simulink model "Test_Memory_Block_Word_VRAM_Get_Pixel"  (Simulink 8.7)
settings: Solver=ode45  StartTime=0.0  StopTime=len  RelTol=1e-3
libraries: Miscellaneous x2, Memory_Blocks_Lib x1
settings Model: Creator=N  LastModifiedBy=Jozko Mrkvicka
settings DataIOCC: LimitDataPoints=off
settings DebuggingCC: UnderspecifiedInitializationDetection=Simplified  MergeDetectMultiDrivingBlocksExec=error
settings HardwareCC: ProdBitPerPointer=64  ProdLargestAtomicFloat=Float  ProdIntDivRoundTo=Zero  ProdEndianess=LittleEndian  ProdHWDeviceType=Intel->x86-64 (Windows64)
settings ModelReferenceCC: PropagateSignalLabelsOutOfModel=on

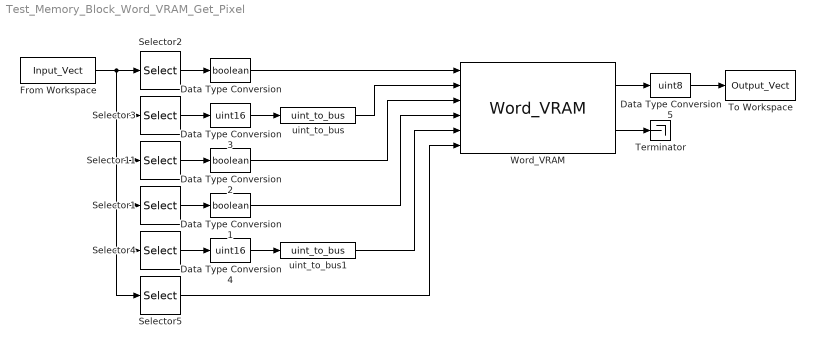
== system Test_Memory_Block_Word_VRAM_Get_Pixel ==
  Data Type Conversion : DataTypeConversion  OutDataTypeStr=boolean
  Data Type Conversion1 : DataTypeConversion  OutDataTypeStr=boolean
  Data Type Conversion2 : DataTypeConversion  OutDataTypeStr=boolean
  Data Type Conversion3 : DataTypeConversion  OutDataTypeStr=uint16
  Data Type Conversion4 : DataTypeConversion  OutDataTypeStr=uint16
  Data Type Conversion5 : DataTypeConversion  OutDataTypeStr=uint8
  From Workspace : FromWorkspace  VariableName=Input_Vect  SampleTime=1  Interpolate=off  OutputAfterFinalValue=Holding final value
  Selector1 : Selector  IndexMode=Zero-based  InputPortWidth=6  IndexOptions=Index vector (dialog)  Indices=3  OutputSizes=1
  Selector11 : Selector  IndexMode=Zero-based  InputPortWidth=6  IndexOptions=Index vector (dialog)  Indices=2  OutputSizes=1
  Selector2 : Selector  IndexMode=Zero-based  InputPortWidth=6  IndexOptions=Index vector (dialog)  Indices=0  OutputSizes=1
  Selector3 : Selector  IndexMode=Zero-based  InputPortWidth=6  IndexOptions=Index vector (dialog)  Indices=1  OutputSizes=1
  Selector4 : Selector  IndexMode=Zero-based  InputPortWidth=6  IndexOptions=Index vector (dialog)  Indices=4  OutputSizes=1
  Selector5 : Selector  IndexMode=Zero-based  InputPortWidth=6  IndexOptions=Index vector (dialog)  Indices=5  OutputSizes=1
  Terminator : Terminator
  To Workspace : ToWorkspace  VariableName=Output_Vect  SampleTime=1
  Word_VRAM : Memory_Blocks_Lib/Memory_Blocks_Lib/Word_VRAM
  uint_to_bus : Miscellaneous/uint_to_bus
  uint_to_bus1 : Miscellaneous/uint_to_bus
  wires:
  Word_VRAM/1 -> Data Type Conversion5/1
  Data Type Conversion5/1 -> To Workspace/1
  Selector11/1 -> Data Type Conversion2/1
  Selector2/1 -> Data Type Conversion/1
  Selector1/1 -> Data Type Conversion1/1
  From Workspace/1 -> Selector3/1, Selector4/1, Selector5/1, Selector1/1, Selector11/1, Selector2/1
  Data Type Conversion/1 -> Word_VRAM/1
  Selector3/1 -> Data Type Conversion3/1
  Data Type Conversion3/1 -> uint_to_bus/1
  Data Type Conversion2/1 -> Word_VRAM/3
  Word_VRAM/2 -> Terminator/1
  uint_to_bus/1 -> Word_VRAM/2
  uint_to_bus1/1 -> Word_VRAM/5
  Selector5/1 -> Word_VRAM/6
  Data Type Conversion1/1 -> Word_VRAM/4
  Data Type Conversion4/1 -> uint_to_bus1/1
  Selector4/1 -> Data Type Conversion4/1
